simulink model "relayswitchexample"  (R2024b)
settings: Solver=VariableStepAuto  StartTime=0.0  StopTime=10.0  RelTol=1e-3
libraries: simulink x1
settings Model: Creator=ada09  LastModifiedBy=ada09

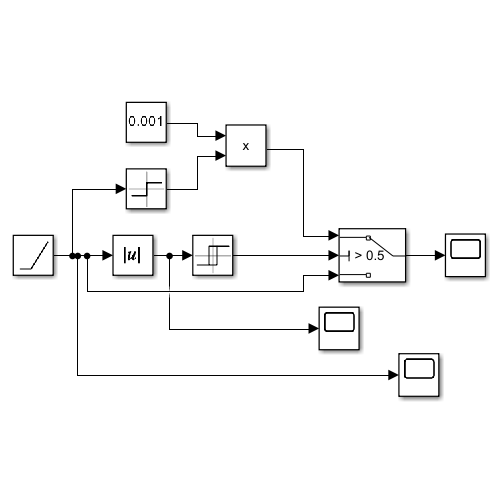
[thumbnail: Simulink's stored preview of the top-level diagram]
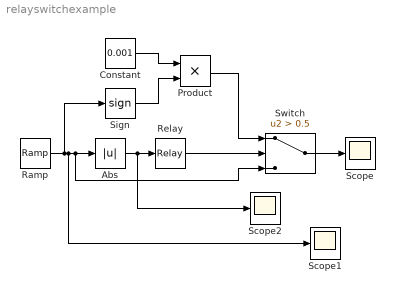
== system relayswitchexample ==
  Abs : Abs  SaturateOnIntegerOverflow=off
  Constant : Constant  Value=0.001
  Product : Product
  Ramp : simulink/Sources/Ramp  slope=1  start=0  InitialOutput=-1
  Relay : Relay  OnSwitchValue=0.001  OffSwitchValue=0
  Scope : Scope
  Scope1 : Scope
  Scope2 : Scope
  Sign : Signum
  Switch : Switch  Criteria=u2 > Threshold  Threshold=0.5  SaturateOnIntegerOverflow=off  InputSameDT=off
  wires:
  Ramp/1 -> Sign/1, Scope1/1, Switch/3, Abs/1
  Abs/1 -> Scope2/1, Relay/1
  Constant/1 -> Product/1
  Sign/1 -> Product/2
  Product/1 -> Switch/1
  Relay/1 -> Switch/2
  Switch/1 -> Scope/1
